simulink model "cs_proj_ol_step"  (R2021b)
settings: Solver=ode4  StartTime=0.0  StopTime=100.0  FixedStep=0.001  RelTol=1e-3
settings Model: Creator=shash  LastModifiedBy=shash
settings DataIOCC: ReturnWorkspaceOutputs=off

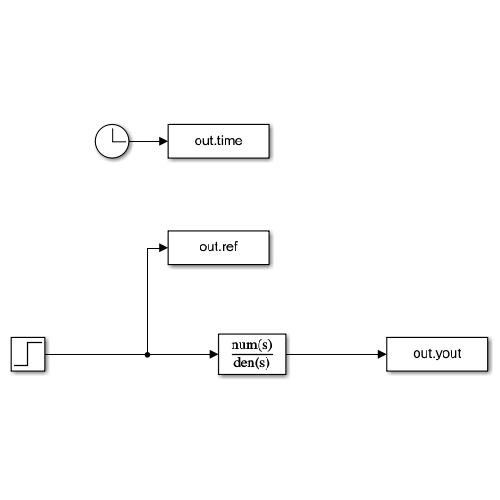
[thumbnail: Simulink's stored preview of the top-level diagram]
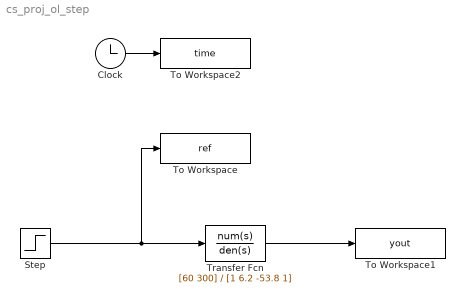
== system cs_proj_ol_step ==
  Clock : Clock
  Step : Step  SampleTime=0
  To Workspace : ToWorkspace  VariableName=ref  SampleTime=-1
  To Workspace1 : ToWorkspace  VariableName=yout  SampleTime=-1
  To Workspace2 : ToWorkspace  VariableName=time  SampleTime=-1
  Transfer Fcn : TransferFcn  Numerator=[60 300]  Denominator=[1 6.2 -53.8 1]
  wires:
  Step/1 -> To Workspace/1, Transfer Fcn/1
  Transfer Fcn/1 -> To Workspace1/1
  Clock/1 -> To Workspace2/1
